simulink model "Bc"  (R2020a)
settings: Solver=VariableStepAuto  StartTime=0.0  StopTime=10.0  RelTol=1e-3
settings Model: Creator=Pranshu  LastModifiedBy=Pranshu

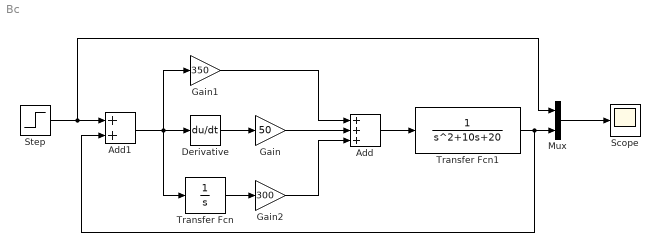
== system Bc ==
  Add : Sum  Inputs=+++
  Add1 : Sum
  Derivative : Derivative
  Gain : Gain  Gain=50
  Gain1 : Gain  Gain=350
  Gain2 : Gain  Gain=300
  Mux : Mux  Inputs=2
  Scope : Scope
  Step : Step  Time=0  SampleTime=0
  Transfer Fcn : TransferFcn  Denominator=[1 0]
  Transfer Fcn1 : TransferFcn  Denominator=[1 10 20]
  wires:
  Transfer Fcn1/1 -> Add1/2, Mux/2
  Derivative/1 -> Gain/1
  Transfer Fcn/1 -> Gain2/1
  Step/1 -> Add1/1, Mux/1
  Add/1 -> Transfer Fcn1/1
  Gain/1 -> Add/2
  Gain1/1 -> Add/1
  Gain2/1 -> Add/3
  Mux/1 -> Scope/1
  Add1/1 -> Transfer Fcn/1, Gain1/1, Derivative/1
